simulink model "Model_References"  (R2024b)
settings: Solver=VariableStepAuto  StartTime=0.0  StopTime=10.0  RelTol=1e-3
InitFcn:
  | J =0.01;
  | b = 0.1;
  | K = 0.01;
  | R = 1;
  | kb =0.01;
  | L = 0.5;
  | Kp=550;
  | ki = 500;
  | Ts = 0.01;
  | Kd =0.01;
settings Model: Creator=chall  LastModifiedBy=Sagar

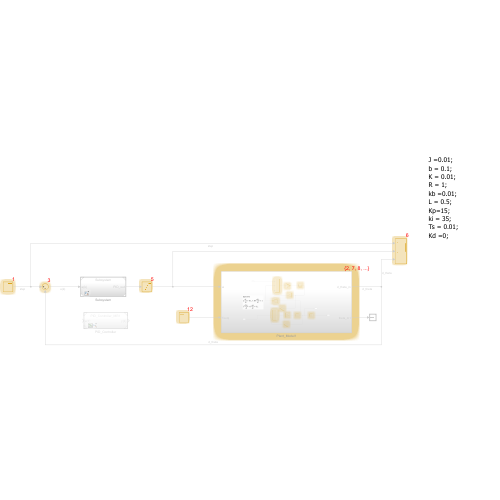
[thumbnail: Simulink's stored preview of the top-level diagram]
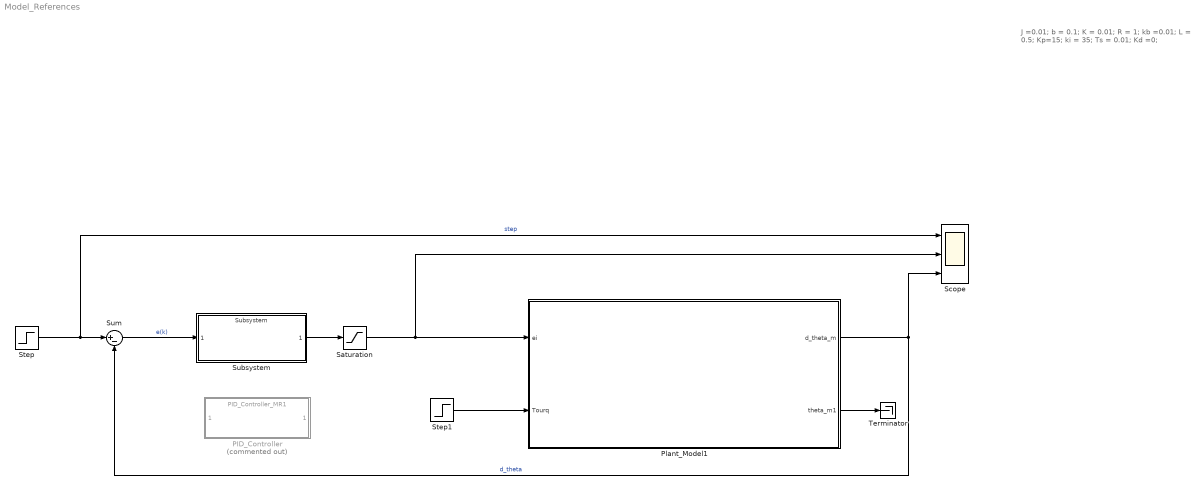
== system Model_References ==
  note: J =0.01;
      | b = 0.1;
      | K = 0.01;
      | R = 1;
      | kb =0.01;
      | L = 0.5;
      | Kp=15;
      | ki = 35;
      | Ts = 0.01;
      | Kd =0;
  PID_Controller : ModelReference  Commented=on  ModelNameDialog=PID_Controller_MR1  SimulationMode=Normal  ModelReferenceVersion=1.4
  Plant_Model1 : Subsystem
  Saturation : Saturate  UpperLimit=25  LowerLimit=-25
  Scope : Scope  NumInputPorts=3
  Step : Step  SampleTime=0
  Step1 : Step  Time=5  After=-0.01  SampleTime=0
  Subsystem : ModelReference  ModelNameDialog=Subsystem  SimulationMode=Normal  ModelReferenceVersion=1.5
  Sum : Sum  Inputs=|+-
  Terminator : Terminator
  wires:
  Step/1 -> Scope/1, Sum/1  "step"
  Plant_Model1/1(d_theta_m) -> Sum/2, Scope/3  "d_theta"
  Plant_Model1/2(theta_m1) -> Terminator/1
  Saturation/1 -> Scope/2, Plant_Model1/1(ei)
  Step1/1 -> Plant_Model1/2(Tourq)
  Sum/1 -> Subsystem/1  "e(k)"
  Subsystem/1 -> Saturation/1

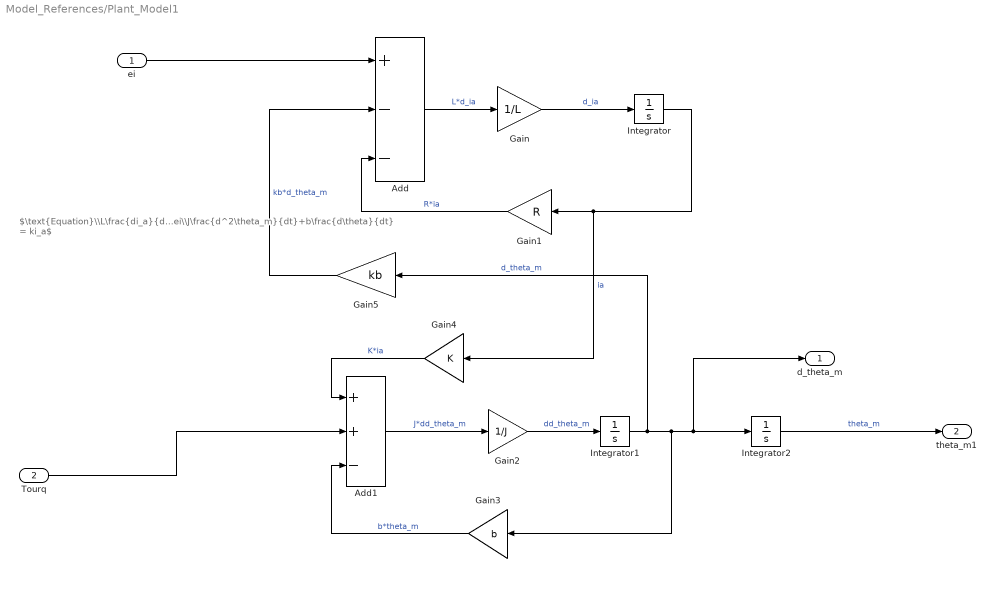
== system Model_References/Plant_Model1 ==
  note: $\text{Equation}\\L\frac{di_a}{dt}+Ri_a+Kb\frac{d\theta_m}{dt}=ei\\J\frac{d^2\theta_m}{dt}+b\frac{d\theta}{dt} = ki_a$
  ei : Inport
  Tourq : Inport  Port=2
  Add : Sum  Inputs=+--
  Add1 : Sum  Inputs=++-
  Gain : Gain  Gain=1/L
  Gain1 : Gain  Gain=R
  Gain2 : Gain  Gain=1/J
  Gain3 : Gain  Gain=b
  Gain4 : Gain  Gain=K
  Gain5 : Gain  Gain=kb
  Integrator : Integrator
  Integrator1 : Integrator
  Integrator2 : Integrator
  d_theta_m : Outport
  theta_m1 : Outport  Port=2
  wires:
  Tourq/1 -> Add1/2
  Integrator2/1 -> theta_m1/1  "theta_m"
  Gain5/1 -> Add/2  "kb*d_theta_m"
  Gain4/1 -> Add1/1  "K*ia"
  Add1/1 -> Gain2/1  "J*dd_theta_m"
  Gain1/1 -> Add/3  "R*ia"
  Add/1 -> Gain/1  "L*d_ia"
  Gain/1 -> Integrator/1  "d_ia"
  ei/1 -> Add/1
  Integrator/1 -> Gain4/1, Gain1/1  "ia"
  Integrator1/1 -> Gain3/1, Integrator2/1, d_theta_m/1, Gain5/1  "d_theta_m"
  Gain2/1 -> Integrator1/1  "dd_theta_m"
  Gain3/1 -> Add1/3  "b*theta_m"
